simulink model "lr5"  (R2022a)
settings: Solver=FixedStepAuto  StartTime=0.0  StopTime=100  FixedStep=1e-2  RelTol=1e-3
libraries: instrumentseriallib x2
settings Model: Creator=User  LastModifiedBy=User

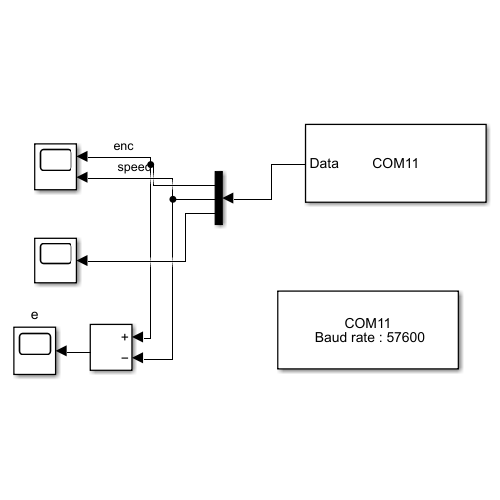
[thumbnail: Simulink's stored preview of the top-level diagram]
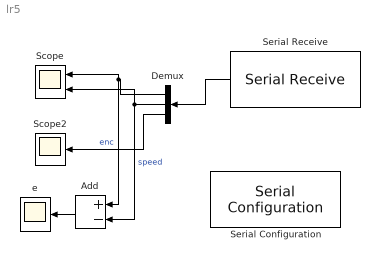
== system lr5 ==
  Add : Sum  Inputs=+-
  Demux : Demux  Outputs=3
  Scope : Scope  NumInputPorts=2
  Scope2 : Scope
  Serial Configuration : instrumentseriallib/Serial Configuration  Priority=-200000  PortSel=COM11  Port=COM11  ComPort=COM11  BaudRate=57600  DataBits=8  Parity=none  StopBits=1  ByteOrder=little-endian  FlowControl=none  Timeout=10  SimulateUsing=Interpreted execution  BlockInModel=on  aMode=1
      settings: SourceProductBaseCode=OT,IC,MT
  Serial Receive : instrumentseriallib/Serial Receive  Priority=1  PortSel=COM11  Port=COM11  ComPort=COM11  DataType=single  SaveDataType=uint8  ToggleHeader=on  Header='rrrr'  ToggleTerminator=on  Terminator=Custom terminator  CustomTerminator='nnnn'  InputFormat=Row major  ToggleDataSize=on  DataSize=[3]  EnableBlockingMode=on  ActionDataUnavailable=Output custom value  ActionWhenDataUnavailable=Output custom value  CustomValue=-1  SampleTime=0.01  SimulateUsing=Interpreted execution  BlockInModel=on  aMode=1
      settings: SourceProductBaseCode=OT,IC,MT
  e : Scope
  wires:
  Serial Receive/1 -> Demux/1
  Demux/1 -> Add/1, Scope/1  "enc"
  Demux/2 -> Add/2, Scope/2  "speed"
  Demux/3 -> Scope2/1
  Add/1 -> e/1
